simulink model "rl"  (R2020b)
settings: Solver=VariableStepAuto  StartTime=0.0  StopTime=0.2  RelTol=1e-3
model workspace (MAT data in the model file):
  R = 2
  a = 220
  freq = 314.16
values from neighbouring files (symbols this model uses):
  E = 10    [task1.m]
  L = 0.05    [task1.m]
settings Model: OrderedModelArguments=off  Creator=axelfroborg  LastModifiedBy=axelfroborg
settings DataIOCC: TimeSaveName=tdc

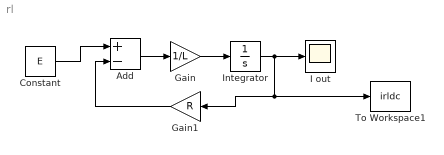
== system rl ==
  Add : Sum  Inputs=+-
  Constant : Constant  Value=E
  Gain : Gain  Gain=1/L
  Gain1 : Gain  Gain=R
  I out : Scope
  Integrator : Integrator
  To Workspace1 : ToWorkspace  VariableName=irldc  SampleTime=-1
  wires:
  Integrator/1 -> Gain1/1, To Workspace1/1, I out/1
  Add/1 -> Gain/1
  Gain/1 -> Integrator/1
  Gain1/1 -> Add/2
  Constant/1 -> Add/1
